simulink model "V5_SUB_Geschalteter_Eingang_Validierung"  (R2022b)
settings: Solver=VariableStepAuto  StartTime=0.0  StopTime=10.0  RelTol=1e-3
settings Model: Creator=JSCHB  LastModifiedBy=JSCHB

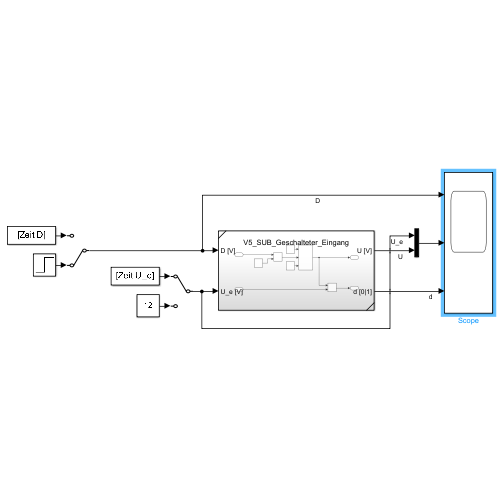
[thumbnail: Simulink's stored preview of the top-level diagram]
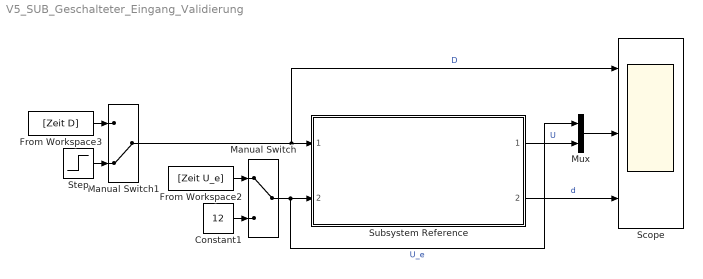
== system V5_SUB_Geschalteter_Eingang_Validierung ==
  Constant1 : Constant  Value=12
  From Workspace2 : FromWorkspace  VariableName=[Zeit U_e]
  From Workspace3 : FromWorkspace  VariableName=[Zeit D]
  Manual Switch : ManualSwitch
  Manual Switch1 : ManualSwitch  CurrentSetting=0
  Mux : Mux  Inputs=2
  Scope : Scope  NumInputPorts=3
  Step : Step  Before=7  After=8  SampleTime=0
  Subsystem Reference : Subsystem  ReferencedSubsystem=V5_SUB_Geschalteter_Eingang
  wires:
  From Workspace2/1 -> Manual Switch/1
  Constant1/1 -> Manual Switch/2
  Manual Switch/1 -> Mux/1, Subsystem Reference/2  "U_e"
  From Workspace3/1 -> Manual Switch1/1
  Step/1 -> Manual Switch1/2
  Manual Switch1/1 -> Scope/1, Subsystem Reference/1  "D"
  Subsystem Reference/2 -> Scope/3  "d"
  Mux/1 -> Scope/2
  Subsystem Reference/1 -> Mux/2  "U"
